simulink model "SingleRoom"  (R2020b)
settings: Solver=ode45  StartTime=0  StopTime=31449600  FixedStep=0.3  MaxStep=900  RelTol=1e-6
values from neighbouring files (symbols this model uses):
  P = getParameters('T_s',15,'Hp_val',Hp_val_flo,'PeriodicOccupancy',true)    [run_ident.m]    (also in run_sim.m = getParameters('T_s',15,'PeriodicOccupancy',false))
settings Model: Creator=jpatsch  LastModifiedBy=fpaschke
settings DebuggingCC: UnderSpecifiedDimensionMsg=warning  ArithmeticOperatorsInVariantConditions=warning
settings SFSimCC: CustomCodeUndefinedFunction=UseInterfaceOnly

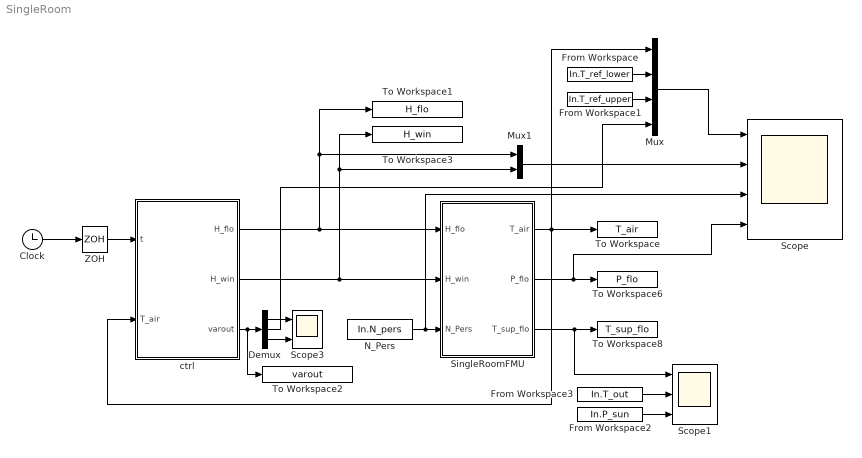
== system SingleRoom ==
  Clock : Clock
  Demux : Demux  Outputs=3
  From Workspace : FromWorkspace  VariableName=In.T_ref_lower  SampleTime=P.T_s*60
  From Workspace1 : FromWorkspace  VariableName=In.T_ref_upper  SampleTime=P.T_s*60
  From Workspace2 : FromWorkspace  VariableName=In.P_sun  SampleTime=P.T_s*60
  From Workspace3 : FromWorkspace  VariableName=In.T_out  SampleTime=P.T_s*60
  Mux : Mux
  Mux1 : Mux  Inputs=2
  N_Pers : FromWorkspace  VariableName=In.N_pers  OutDataTypeStr=double  SampleTime=P.T_s*60
  Scope : Scope  NumInputPorts=4
  Scope1 : Scope  NumInputPorts=3
  Scope3 : Scope  NumInputPorts=2
  SingleRoomFMU : Subsystem
  To Workspace : ToWorkspace  VariableName=T_air  SaveFormat=Timeseries  SampleTime=P.T_s*60
  To Workspace1 : ToWorkspace  VariableName=H_flo  SaveFormat=Timeseries  SampleTime=P.T_s*60
  To Workspace2 : ToWorkspace  VariableName=varout  SaveFormat=Timeseries  SampleTime=P.T_s*60
  To Workspace3 : ToWorkspace  VariableName=H_win  SaveFormat=Timeseries  SampleTime=P.T_s*60
  To Workspace6 : ToWorkspace  VariableName=P_flo  SaveFormat=Timeseries  SampleTime=P.T_s*60
  To Workspace8 : ToWorkspace  VariableName=T_sup_flo  SaveFormat=Timeseries  SampleTime=P.T_s*60
  ZOH : ZeroOrderHold  SampleTime=P.T_s*60
  ctrl : MATLAB Function  TreatAsAtomicUnit=on
  wires:
  ZOH/1 -> ctrl/1(t)
  Clock/1 -> ZOH/1
  Mux/1 -> Scope/1
  SingleRoomFMU/1(T_air) -> To Workspace/1, Mux/1, ctrl/2(T_air)
  N_Pers/1 -> Scope/3, SingleRoomFMU/3(N_Pers)
  SingleRoomFMU/2(P_flo) -> Scope/4, To Workspace6/1
  ctrl/2(H_win) -> SingleRoomFMU/2(H_win), To Workspace3/1, Mux1/2
  ctrl/1(H_flo) -> SingleRoomFMU/1(H_flo), To Workspace1/1, Mux1/1
  Mux1/1 -> Scope/2
  SingleRoomFMU/3(T_sup_flo) -> Scope1/1, To Workspace8/1
  From Workspace1/1 -> Mux/3
  From Workspace/1 -> Mux/2
  ctrl/3(varout) -> To Workspace2/1, Demux/1
  Demux/1 -> Scope3/1
  Demux/2 -> Mux/4
  From Workspace3/1 -> Scope1/2
  From Workspace2/1 -> Scope1/3
  Demux/3 -> Scope3/2

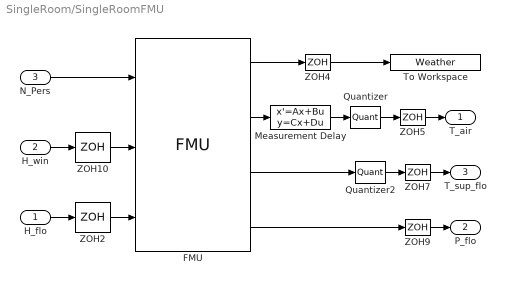
== system SingleRoom/SingleRoomFMU ==
  H_flo : Inport
  H_win : Inport  Port=2
  N_Pers : Inport  Port=3
  FMU : FMU  FMUName=SingleRoom.fmu  FMUDebugLogging=on  FMUMode=ModelExchange  system=struct('p_ambient',101325,'T_ambient',293.15,'g',9.80665,'m_flow_start',0,'eps_m_flow',0.0001,'dp_small',1,'m_flow_small',0.01)  h_room=3  h_win=2  w_win=6  T_room_nominal=295.15  dp_valve_flo_nominal=100  p_sink_flo=100000  Tsup_flo_cool=18  T_cool_startday=120  T_cool_endday=273  Roo=struct('lat',0.91664692314742,'conExtWin',[struct('glaSys',struct('haveControllableWindow',boolean(false)),'win',struct('glaUns',struct('glass',[struct('T0',293.15),struct('T0',293.15)],'gas',[struct('T0',293.15)]),'glaSha',struct('glass',[struct('T0',293.15),struct('T0',293.15)],'gas',[struct('T0',293.15)])))],'hIntFixed',3.0,'hExtFixed',10.0,'bouConExtWin',struct('conPar',[struct('ove',struct('dep',0),'sidFin',struct('dep',0))],'HDifTil',[struct('rho',0.2,'add',struct('k1',1,'k2',1))],'conExtWin',[struct('radOut',struct('T0',293.15),'shaRad',struct('T0',293.15))]),'air',struct('convConWin',[struct('conSha',struct('k',1))]),'p_start',101325,'T_start',293.15,'X_start',[0.01,0.99],'shaRad',[struct('T0',293.15)])  WeaData=struct('pAtm',101325,'TDryBul',293.15,'TDewPoi',283.15,'TBlaSky',273.15,'relHum',0.5,'winSpe',1,'winDir',1.0,'HInfHor',0.0,'ceiHei',20000,'totSkyCov',0.5,'opaSkyCov',0.5)  WallNorth=struct('T_a_start',293.15,'T_b_start',293.15)  WallEast=struct('T_a_start',293.15,'T_b_start',293.15)  WallSouth=struct('T_a_start',293.15,'T_b_start',293.15)  Ceiling=struct('T_a_start',293.15,'T_b_start',293.15)  TemTab=struct('verboseRead',boolean(true),'columns',[int32(2),int32(3),int32(4),int32(5),int32(6)],'offset',[0],'startTime',0,'timeEvents',int32(1))  Ceil=struct('absIR_a',0.9,'absIR_b',0.9,'absSol_a',0.5,'absSol_b',0.5,'roughness_a',int32(3))  Iw=struct('absIR_a',0.9,'absIR_b',0.9,'absSol_a',0.5,'absSol_b',0.5,'roughness_a',int32(3))  Ow=struct('absIR_a',0.9,'absIR_b',0.9,'absSol_a',0.5,'absSol_b',0.5,'roughness_a',int32(3))  FloHeat=struct('sysTyp',int32(2),'T_a_start',293.15,'T_b_start',293.15,'p_start',300000,'T_start',293.15,'X_start',[1],'mSenFac',1,'deltaM',0.1,'sla',struct('mSenFac',1))  Val=struct('deltaM',0.02,'rhoStd',995.586,'riseTime',120,'y_start',1,'l',0.0001,'R',50,'delta0',0.01)  SinFlo=struct('X',[1])  Sou=struct('X',[1])  HcvFlo=struct('m',1.1,'TRoo_nominal',293.15,'TOut_nominal',258.15,'dTOutHeaBal',0)  Flo=struct('absIR_a',0.9,'absIR_b',0.9,'absSol_a',0.5,'absSol_b',0.5,'roughness_a',int32(3))  Pip=struct('dOut',0.025,'d',983,'k',0.35)  DeltaTflo=struct('k1',1,'k2',-1)  Cw=struct('k',4.184)  Win_2=struct('glass',[struct('x_2',0.003,'k',1.0,'tauSol',[0.834],'rhoSol_a',[0.075],'rhoSol_b',[0.075],'tauIR',0.0,'absIR_a',0.84,'absIR_b',0.84),struct('x_2',0.003,'k',1.0,'tauSol',[0.834],'rhoSol_a',[0.075],'rhoSol_b',[0.075],'tauIR',0.0,'absIR_a',0.84,'absIR_b',0.84)],'gas',[struct('x_2',0.0127,'a_k',0.002873,'b_k',7.76E-05,'a_mu',3.723E-06,'b_mu',4.94E-08,'a_c',1002.737,'b_c',0.012324,'MM',0.02897,'P0',101325.0)],'shade',struct('tauSol_a',0.1,'tauSol_b',0.1,'rhoSol_a',0.8,'rhoSol_b',0.8,'absIR_a',0.84,'absIR_b',0.84,'tauIR_a',0.0,'tauIR_b',0.0),'UFra',1.4,'absIRFra',0.8,'absSolFra',0.5)  mask(SingleRoom [Model Exchange, v2.0]){}
      settings: MultiThreadCoSim=off
      mask Display:
      | disp('SingleRoom');
      | port_label('output',1,'Wb');
      | port_label('output',2,'T_room');
      | port_label('output',3,'T_sup_flo');
      | port_label('output',4,'P_flo');
      | port_label('input',1,'N_Pers');
      | port_label('input',2,'H_win');
      | port_label('input',3,'H_flo');
  Measurement Delay : StateSpace  A=-eye(1)./(P.T_sens*60)  B=eye(1)./(P.T_sens*60)  C=eye(1)  D=zeros(1)  InitialCondition=20*ones(1,1)
  Quantizer : Quantizer  QuantizationInterval=P.Q_int
  Quantizer2 : Quantizer  QuantizationInterval=P.Q_int
  To Workspace : ToWorkspace  VariableName=Weather  SaveFormat=Timeseries  SampleTime=P.T_s*60
  ZOH{2,4..5,7,9..10} (6 alike) : ZeroOrderHold  SampleTime=P.T_s*60
  T_air : Outport
  P_flo : Outport  Port=2
  T_sup_flo : Outport  Port=3
  wires:
  Measurement Delay/1 -> Quantizer/1
  H_flo/1 -> ZOH2/1
  FMU/2 -> Measurement Delay/1
  FMU/1 -> ZOH4/1
  ZOH4/1 -> To Workspace/1
  N_Pers/1 -> FMU/1
  Quantizer/1 -> ZOH5/1
  ZOH5/1 -> T_air/1
  ZOH7/1 -> T_sup_flo/1
  Quantizer2/1 -> ZOH7/1
  ZOH9/1 -> P_flo/1
  FMU/4 -> ZOH9/1
  H_win/1 -> ZOH10/1
  ZOH10/1 -> FMU/2
  ZOH2/1 -> FMU/3
  FMU/3 -> Quantizer2/1

== matlab function SingleRoom/ctrl ==
  data: t input size=1; T_air input size=1; H_flo output size=1 [0..1]; H_win output size=1 [0..1]; varout output size=3
function [H_flo, H_win, varout] = ctrl(t,T_air)
%Calls controller function.

H_flo = NaN;
H_win = NaN;
varout = NaN(3,1);
coder.extrinsic('ctrl_fun');
[H_flo, H_win, varout] = ctrl_fun(t,T_air);
end
